simulink model "PI_UDP_Recieve"  (Simulink 10.0)
settings: Solver=FixedStepAuto  StartTime=0.0  StopTime=inf  RelTol=1e-3  EnableMultiTasking=on
libraries: simulink x1, raspberrypilib x1, logitechG29 x1, embdlinuxlib x1
settings Model: LogicAnalyzerSignalOrdering=48fb4b40-4eda-496c-aded-dfb39eef3e7e,bd087c1e-8b80-42f3-8cd6-3d9603fa049d,db1d0dea-daf4-49a5-865c-471e128446e0  Creator=fredd  LastModifiedBy=FRED-Surface  SimulationMode=external
settings Model: SuppressorTable=|
  | <?xml version="1.0" encoding="UTF-8" standalone="yes" ?>
  | <!DOCTYPE boost_serialization>
  | <boost_serialization signature="serialization::archive" version="15">
  | <DiagnosticSuppressor class_id="0" tracking_level="0" version="6">
  | 	<Table class_id="1" tracking_level="0" version="0">
  | 		<count>1</count>
  | 		<bucket_count>8</bucket_count>
  | 		<item_version>0</item_version>
  | 		<item class_id="2" tracking_level="0" version="0">
  | 			<first class_id="3" tracking_level="0" version="6">
  | 				<Source class_id="4" tracking_level="0" version="0">
  | 					<count>1</count>
  | 					<item_version>0</item_version>
  | 					<item>PI_UDP_Recieve/Counter Limited</item>
  | 				</Source>
  | 			</first>
  | 			<second class_id="5" tracking_level="0" version="6">
  | 				<SuppressedData class_id="6" tracking_level="0" version="0">
  | 					<count>2</count>
  | 					<bucket_count>8</bucket_count>
  | 					<item_version>0</item_version>
  | 					<item class_id="7" tracking_level="0" version="0">
  | 						<first class_id="8" tracking_level="0" version="6">
  | 							<ID>Simulink:DataType:WarningOverFlowDetected</ID>
  | 							<Cause>
  | 								<Source>
  | 									<count>0</count>
  | 									<item_version>0</item_version>
  | 								</Source>
  | 							</Cause>
  | 						</first>
  | 						<second class_id="9" tracking_level="0" version="6">
  | 							<Comment></Comment>
  | 							<User></User>
  | 							<LastModified class_id="10" tracking_level="0" version="0">
  | 								<ptime_date class_id="11" tracking_level="0" version="0">
  | 									<date>20160608</date>
  | 								</ptime_date>
  | 								<ptime_time_duration class_id="12" tracking_level="0" version="0">
  | 									<is_special>0</is_special>
  | 									<time_duration_hours>15</time_duration_hours>
  | 									<time_duration_minutes>23</time_duration_minutes>
  | 									<time_duration_seconds>17</time_duration_seconds>
  | 									<time_duration_fractional_seconds>0</time_duration_fractional_seconds>
  | 								</ptime_time_duration>
  | 							</LastModified>
  | 							<SuppressionType>1</SuppressionType>
  | 						</second>
  | 					</item>
  | 					<item>
  | 						<first>
  | 							<ID>SimulinkFixedPoint:util:Overflowoccurred</ID>
  | 							<Cause>
  | 								<Source>
  | 									<count>0</count>
  | 									<item_version>0</item_version>
  | 								</Source>
  | 							</Cause>
  | 						</first>
  | 						<second>
  | 							<Comment></Comment>
  | 							<User></User>
  | 							<LastModified>
  | 								<ptime_date>
  | 									<date>20160608</date>
  | 								</ptime_date>
  | 								<ptime_time_duration>
  | 									<is_special>0</is_special>
  | 									<time_duration_hours>15</time_duration_hours>
  | 									<time_duration_minutes>23</time_duration_minutes>
  | 									<time_duration_seconds>17</time_duration_seconds>
  | 									<time_duration_fractional_seconds>0</time_duration_fractional_seconds>
  | 								</ptime_time_duration>
  | 							</LastModified>
  | 							<SuppressionType>1</SuppressionType>
  | 						</second>
  | 					</item>
  | 				</SuppressedData>
  | 			</second>
  | 		</item>
  | 	</Table>
  | </DiagnosticSuppressor>
  | </boost_serialization>
settings SolverCC: PositivePriorityOrder=on
settings DataIOCC: SaveFormat=Dataset  ReturnWorkspaceOutputs=on
settings OptimizationCC: EnhancedBackFolding=on  PassReuseOutputArgsAs=Individual arguments  ZeroExternalMemoryAtStartup=off  ZeroInternalMemoryAtStartup=off  LifeSpan=auto  MaxStackSize=64  OptimizeBlockOrder=speed  DifferentSizesBufferReuse=on  OptimizationCustomize=off  EfficientTunableParamExpr=on
settings DebuggingCC: UnderspecifiedInitializationDetection=Simplified  MergeDetectMultiDrivingBlocksExec=error  ParameterTunabilityLossMsg=error  SFUnexpectedBacktrackingDiag=error  SFNoUnconditionalDefaultTransitionDiag=error  SFExecutionAtInitializationDiag=warning  ArithmeticOperatorsInVariantConditions=error
settings HardwareCC: ProdLargestAtomicInteger=Long  ProdLargestAtomicFloat=Double  ProdIntDivRoundTo=Zero  ProdEndianess=LittleEndian  ProdLongLongMode=on  ProdHWDeviceType=ARM Compatible->ARM Cortex
settings ModelReferenceCC: PropagateSignalLabelsOutOfModel=on
settings SFSimCC: SimUseLocalCustomCode=on  CustomCodeUndefinedFunction=FilterOut
settings SFSimCC: SimUserSources=|
  | Window.h
  | Xinput.h
settings RTWCC: Description=Embedded Coder  SystemTargetFile=ert.tlc  HardwareBoard=Raspberry Pi  TLCOptions="-aInlineSetEventsForThisBaseRateFcn=TLC_FALSE -aSuppressMultiTaskScheduler=TLC_FALSE  -aRateBasedStepFcn=0"  TemplateMakefile=ert_default_tmf  GenerateReport=on  RTWUseLocalCustomCode=on  Toolchain=GNU GCC Raspberry Pi  BuildConfiguration=Faster Runs  IncludeHyperlinkInReport=on  LaunchReport=on  GenerateTraceInfo=on  GenerateTraceReport=on  GenerateTraceReportSl=on  GenerateTraceReportSf=on  GenerateTraceReportEml=on
settings MATStruct: className=codertarget.tools.BuildHook  argsTopModelOnly=[]  excludedModels=[]  includeReferencedModels=on  includeTopModel=on  enabled=on  UseCoderTarget=[1.0]  TargetHardware=Raspberry Pi  RTOS=Linux  RTOSBaseRateTaskPriority=40  DetectTaskOverruns=[0.0]  Scheduler_interrupt_source=[0.0]  DataVersion=2016.02  IPAddress=codertarget.raspi.getDeviceAddress  Port=17725  Verbose=[0.0]  RunInBackground=[0.0]  Configuration=XCP on TCP/IP  signalBufferSize=[1000000.0]  Running=on  DeviceAddress=192.168.137.229  Username=pi  Password=Raspberry1  BuildDir=/home/pi  BuildAction=Build and run  RunOnBoot=[0.0]  SPI0CE0BusSpeed=1000  SPI0CE1BusSpeed=1000  CANBusSpeed=500  CANOscillatorFrequency=16  InterruptPin=12  AllowAllFilter=[1.0]  Buffer0IDType=Normal  AcceptanceMask0=0  AcceptanceFilter0=255  AcceptanceFilter1=255  Buffer1IDType=Normal  AcceptanceMask1=0  AcceptanceFilter2=255  AcceptanceFilter3=255  AcceptanceFilter4=255  AcceptanceFilter5=255  BrokerAddress=mqtt.thingspeak.com
settings CodeAppCC: ForceParamTrailComments=on  IgnoreCustomStorageClasses=off  OperatorAnnotations=on  SimulinkDataObjDesc=on  SFDataObjDesc=on  InsertBlockDesc=on  StateflowObjectComments=off
settings ERTTargetCC: SupportContinuousTime=on  SupportNonInlinedSFcns=on  SupportVariableSizeSignals=on  ExtMode=on  ExtModeTransport=2  ExtModeStaticAlloc=on  ExtModeMexFile=ext_xcp  ExtModeMexArgs='192.168.0.36' 0 17725  ExtModeIntrfLevel=Level2 - Open
settings ConfigComp: CovMetricSettings=dwe  CovHtmlReporting=off  CovSaveCumulativeToWorkspaceVar=off  CovSaveSingleToWorkspaceVar=off

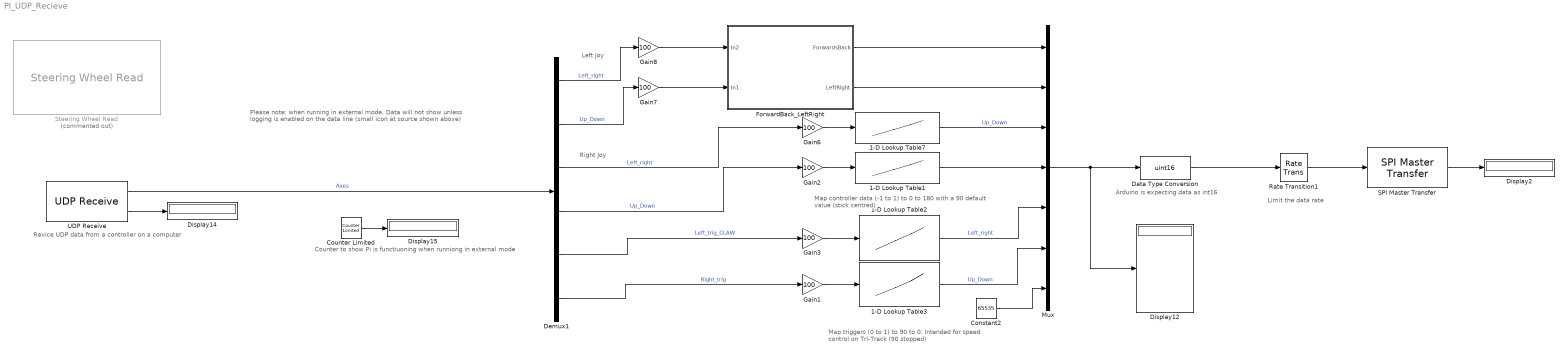
== system PI_UDP_Recieve ==
  note: Please note: when running in external mode, Data will not show unless logging is enabled on the data line (small icon at source shown above)
  note: Limit the data rate
  note: Arduino is expecting data as int16
  note: Map triggers (0 to 1) to 90 to 0. Intended for speed control on Tri-Track (90 stopped)
  note: Map controller data (-1 to 1) to 0 to 180 with a 90 default value (stick centred)
  note: Revice UDP data from a controller on a computer
  note: Counter to show Pi is functiuoning when runniong in external mode
  note: Left Joy
  note: Right Joy
  1-D Lookup Table1 : Lookup_n-D  NumberOfTableDimensions=1  BreakpointsForDimension1=[-100,-50,0,50,100]  BreakpointsForDimension1FirstPoint=0  BreakpointsForDimension1Spacing=1.8  Table=[1000;1120;1280;1750;2000]  ExtrapMethod=Clip  InternalRulePriority=Speed  RndMeth=Simplest  InputSameDT=on
  1-D Lookup Table2 : Lookup_n-D  NumberOfTableDimensions=1  BreakpointsForDimension1=[0,50,100]  BreakpointsForDimension1FirstPoint=0  BreakpointsForDimension1Spacing=1.8  Table=[90,45,0]  ExtrapMethod=Clip  InternalRulePriority=Speed  RndMeth=Simplest  InputSameDT=on
  1-D Lookup Table3 : Lookup_n-D  NumberOfTableDimensions=1  BreakpointsForDimension1=[0,50,100]  BreakpointsForDimension1FirstPoint=0  BreakpointsForDimension1Spacing=1.8  Table=[180,90,0]  ExtrapMethod=Clip  InternalRulePriority=Speed  RndMeth=Simplest  InputSameDT=on
  1-D Lookup Table7 : Lookup_n-D  NumberOfTableDimensions=1  BreakpointsForDimension1=[-100,-50,0,50,100]  BreakpointsForDimension1FirstPoint=0  BreakpointsForDimension1Spacing=1.8  Table=[1000;1120;1280;1750;2000]  ExtrapMethod=Clip  InternalRulePriority=Speed  RndMeth=Simplest  InputSameDT=on
  Constant2 : Constant  Value=65535  OutDataTypeStr=single
  Counter Limited : simulink/Sources/Counter Limited  uplimit=7  tsamp=1
  Data Type Conversion : DataTypeConversion  OutDataTypeStr=uint16  RndMeth=Round  SaturateOnIntegerOverflow=on
  Demux1 : Demux  Outputs=6
  Display{2,12,14..15} (4 alike) : Display
      settings: Format=bank  Decimation=2
  ForwardBack_LeftRight : Subsystem
  Gain{1..3,6..8} (6 alike) : Gain  Gain=100
  Mux : Mux  Inputs=7
  Rate Transition1 : RateTransition  OutPortSampleTime=0.1
  SPI Master Transfer : raspberrypilib/SPI Master Transfer  BoardProperty=Pi 3 Model B+  SPIModule=uint32(0)  Mode=Master  BusSpeed=1000000  Pin=SPI0_CE0  FirstBitToTransfer=Most significant bit (MSB)  ClockMode=0  BlockFunction=Transfer  RegisterAddress=0  OutputDataType=int8  OutputDataLength=1
      settings: SourceProductName=Simulink Support Package for Raspberry Pi Hardware  SourceProductBaseCode=RASPPI
  "Steering Wheel Read " : logitechG29/Steering Wheel Read   Commented=on  sampleTime=-1
      settings: SourceProductName=Simulink Real-Time  SourceProductBaseCode=XP
  UDP Receive : embdlinuxlib/UDP Receive  localURL='0.0.0.0'  localPort=25000  remoteURL='0.0.0.0'  remotePort=-1  recvBufferSize=8192  signalDatatype=single  dims=6  isVarSize=off  showBlockingTime=off  blockingTime=0  sampletime=0.01  blockPlatform=Raspberry Pi
      settings: SourceProductName=Simulink Support Package for Raspberry Pi Hardware  SourceProductBaseCode=RASPPI
  wires:
  UDP Receive/1 -> Demux1/1  "Axes"
  Demux1/2 -> Gain7/1  "Up_Down"
  Demux1/3 -> Gain6/1  "Left_right"
  Demux1/4 -> Gain2/1  "Up_Down"
  Demux1/5 -> Gain3/1  "Left_trig_CLAW"
  Demux1/6 -> Gain1/1  "Right_trig"
  Demux1/1 -> Gain8/1  "Left_right"
  1-D Lookup Table3/1 -> Mux/6  "Up_Down"
  1-D Lookup Table1/1 -> Mux/4
  Gain2/1 -> 1-D Lookup Table1/1
  Gain3/1 -> 1-D Lookup Table2/1
  UDP Receive/2 -> Display14/1
  Counter Limited/1 -> Display15/1
  Gain1/1 -> 1-D Lookup Table3/1
  SPI Master Transfer/1 -> Display2/1
  1-D Lookup Table2/1 -> Mux/5  "Left_right"
  Rate Transition1/1 -> SPI Master Transfer/1
  Data Type Conversion/1 -> Rate Transition1/1
  Constant2/1 -> Mux/7
  Mux/1 -> Data Type Conversion/1, Display12/1
  Gain6/1 -> 1-D Lookup Table7/1
  1-D Lookup Table7/1 -> Mux/3  "Up_Down"
  Gain7/1 -> ForwardBack_LeftRight/2(In1)
  ForwardBack_LeftRight/1(ForwardsBack) -> Mux/1
  ForwardBack_LeftRight/2(LeftRight) -> Mux/2
  Gain8/1 -> ForwardBack_LeftRight/1(In2)

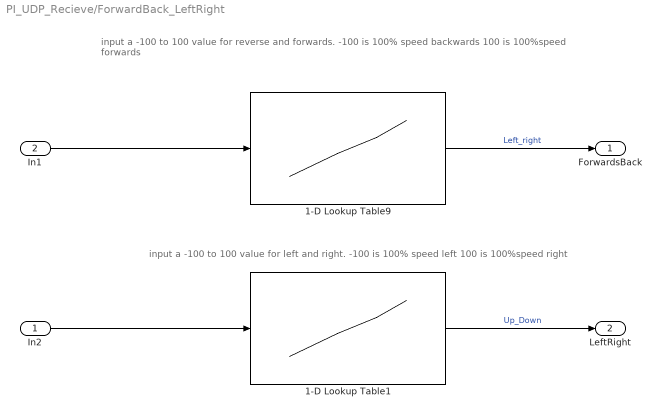
== system PI_UDP_Recieve/ForwardBack_LeftRight ==
  note: input a -100 to 100 value for reverse and forwards. -100 is 100% speed backwards 100 is 100%speed forwards
  note: input a -100 to 100 value for left and right. -100 is 100% speed left 100 is 100%speed right
  In2 : Inport
  In1 : Inport  Port=2
  1-D Lookup Table1 : Lookup_n-D  NumberOfTableDimensions=1  BreakpointsForDimension1=[-100,-50,0,50,100]  BreakpointsForDimension1FirstPoint=0  BreakpointsForDimension1Spacing=1.8  Table=[2000;1750;1500;1250;1000]  ExtrapMethod=Clip  InternalRulePriority=Speed  RndMeth=Simplest  InputSameDT=on
  1-D Lookup Table9 : Lookup_n-D  NumberOfTableDimensions=1  BreakpointsForDimension1=[-100,-50,0,50,100]  BreakpointsForDimension1FirstPoint=0  BreakpointsForDimension1Spacing=1.8  Table=[1000;1250;1500;1750;2000]  ExtrapMethod=Clip  InternalRulePriority=Speed  RndMeth=Simplest  InputSameDT=on
  ForwardsBack : Outport
  LeftRight : Outport  Port=2
  wires:
  In1/1 -> 1-D Lookup Table9/1
  1-D Lookup Table1/1 -> LeftRight/1  "Up_Down"
  1-D Lookup Table9/1 -> ForwardsBack/1  "Left_right"
  In2/1 -> 1-D Lookup Table1/1
